simulink model "Problem5"  (R2020a)
settings: Solver=VariableStepAuto  StartTime=0.0  StopTime=10.0  RelTol=1e-3
model workspace (MAT data in the model file):
  C = 1e-05
  R = 10
settings Model: Creator=tanu  LastModifiedBy=tanu

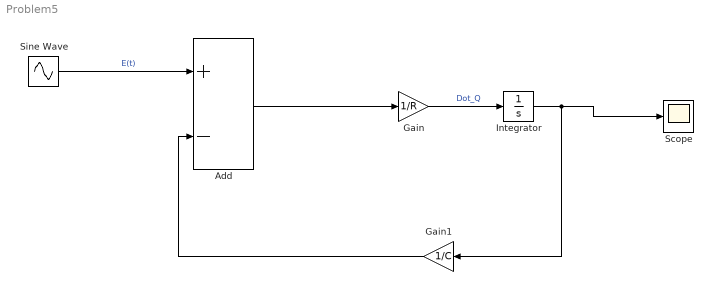
== system Problem5 ==
  Add : Sum  Inputs=+-
  Gain : Gain  Gain=1/R
  Gain1 : Gain  Gain=1/C
  Integrator : Integrator
  Scope : Scope
  Sine Wave : Sin  Amplitude=230  SampleTime=0
  wires:
  Gain/1 -> Integrator/1  "Dot_Q"
  Add/1 -> Gain/1
  Sine Wave/1 -> Add/1  "E(t)"
  Gain1/1 -> Add/2
  Integrator/1 -> Gain1/1, Scope/1
